simulink model "_LongLatDriveline"  (R2020b)
settings: Solver=FixedStepAuto  StartTime=0.0  StopTime=100  FixedStep=0.0005  RelTol=1e-3
InitFcn:
  | load('waypoints.mat');
  | VehicleObj = Simulink.data.dictionary.open('VehicleData.sldd');
  | %dDataSectObj = getSection(myDictionaryObj,'Design Data');
StopFcn:
  | Plot_LateralModelErrorControl;
values from neighbouring files (symbols this model uses):
  A_F = 2.341157    [VehicleData.sldd]
  C_af = 80000.0    [VehicleData.sldd]
  C_ar = 80000.0    [VehicleData.sldd]
  C_d = 0.24    [VehicleData.sldd]
  f = 0.01    [VehicleData.sldd]
  g = 9.81    [VehicleData.sldd]
  h_aero = 0.65    [VehicleData.sldd]
  h_gc = 0.65    [VehicleData.sldd]
  Iz = 2873.0    [VehicleData.sldd]
  lf = 1.1    [VehicleData.sldd]
  lr = 1.58    [VehicleData.sldd]
  m = 2238.932    [VehicleData.sldd]
  Nf = 2.0    [VehicleData.sldd]
  Nr = 2.0    [VehicleData.sldd]
  r_stat = 0.342    [VehicleData.sldd]
  r_w = 0.352    [VehicleData.sldd]
  rho = 1.225    [VehicleData.sldd]
  theta = 0.0    [VehicleData.sldd]
  transGear = 0.1027    [VehicleData.sldd]
  V_wind = 0.0    [VehicleData.sldd]
undefined symbols (not defined in the file or in its folder): sigbuilder_block
settings Model: DataDictionary=VehicleData.sldd  Creator=headl  LastModifiedBy=headl
settings DataIOCC: ReturnWorkspaceOutputs=off  DSMLoggingName=datalog
settings DebuggingCC: SignalRangeChecking=warning
settings SFSimCC: CustomCodeUndefinedFunction=UseInterfaceOnly

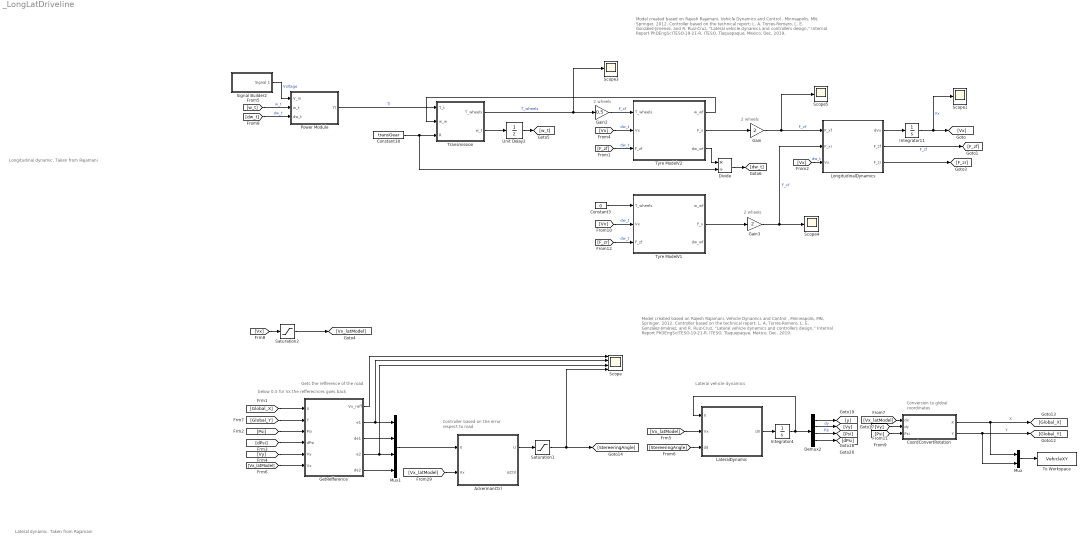
== system _LongLatDriveline ==
  note: below 0.5 for Vx the refferecnces goes back
  note: 2 wheels
  note: Model created based on
      | Rajesh Rajamani, Vehicle Dynamics and Control , Minneapolis, MN, Springer, 2012.
      |
      | Controller based on the technical report:
      | L. A. Torres-Romero, L. E. González-Jiménez, and R. Ruiz-Cruz, “Lateral vehicle dynamics and controllers design,” Internal Report PhDEngScITESO-19-21-R, ITESO, Tlaquepaque, Mexico, Dec. 2019.
  note: Lateral dynamic. Taken from Rajamani
  note: Conversion to global
      | coordinates
  note: Gets the refference of the road
  note: Controller based on the error
      | respect to road
  note: Lateral vehicle dynamics
  note: Longitudinal dynamic. Taken from Rajamani
  note: Model created based on
      | Rajesh Rajamani, Vehicle Dynamics and Control , Minneapolis, MN, Springer, 2012.
      |
      | Controller based on the technical report:
      | L. A. Torres-Romero, L. E. González-Jiménez, and R. Ruiz-Cruz, “Lateral vehicle dynamics and controllers design,” Internal Report PhDEngScITESO-19-21-R, ITESO, Tlaquepaque, Mexico, Dec. 2019.
  note: 2 wheels
  note: 2 wheels
  AckermanCtrl : MATLAB Function  TreatAsAtomicUnit=on
  Constant3 : Constant  Value=0
  Constant30 : Constant  Value=transGear
  CoordConvertRotation : Subsystem
  Demux2 : Demux
  Divide : Product  Inputs=*/
  Gain : Gain  Gain=2
  Gain2 : Gain  Gain=0.5
  Gain3 : Gain  Gain=2
  GetRefference : MATLAB Function  TreatAsAtomicUnit=on
  Integrator11 : Integrator
  Integrator4 : Integrator  InitialCondition=[0;0;-1.574;0.0423]
  LateralDynamic : MATLAB Function  TreatAsAtomicUnit=on
  LongitudinalDynamics : MATLAB Function  TreatAsAtomicUnit=on
  Mux : Mux  Inputs=2
  Mux1 : Mux
  Power Module : Subsystem  Variant=on  VariantControlMode=label  LabelModeActiveChoice=BLDC_Motor
  Saturation1 : Saturate  UpperLimit=pi/4  LowerLimit=-pi/4
  Saturation2 : Saturate  UpperLimit=1000000000  LowerLimit=0.5
  Scope : Scope  NumInputPorts=4
  Scope{1,3..5} (4 alike) : Scope
  Signal Builder2 : Subsystem  Tag=STV Subsys  LoadFcn=sigbuilder_block('load');  StartFcn=sigbuilder_block('start');  StopFcn=sigbuilder_block('stop');  ClipboardFcn=sigbuilder_block('clipboard');  mask(Sigbuilder block){tuvar=[0:10]}
      mask help: Simulink:masks:SigbuilderBlock_MD
      mask init:
      | if ~strcmp(get_param(bdroot(gcbh),'SimulationStatus'),'stopped') tuvar = sigbuilder_block('maskInit'); end
      settings: CopyFcn=sigbuilder_block('copy');  DeleteFcn=sigbuilder_block('delete');  ModelCloseFcn=sigbuilder_block('modelClose');  PreSaveFcn=sigbuilder_block('preSave');  PauseFcn=sigbuilder_block('pause');  ContinueFcn=sigbuilder_block('continue');  NameChangeFcn=sigbuilder_block('namechange');  OpenFcn=sigbuilder_block('open',[5.4 102.6 1141.2 483.6 ]);  CloseFcn=sigbuilder_block('close');
      mask Display: plot(0, 0, 100, 100,[2, 2, 32, 32, 2], [68, 8, 8, 68, 68],[32, 2], [38, 38], [32, 19, 2],[53, 60, 44], [32, 17, 17, 2],[16, 16, 31, 31]);txt = getActiveGroup(gcbh);text(2, 100, txt,'verticalAlignment', 'top');
  To Workspace : ToWorkspace  VariableName=VehicleXY  SampleTime=-1
  Transmission : MATLAB Function  TreatAsAtomicUnit=on
  Tyre ModelV1 : Subsystem
      mask Display: image('D:\Users\headl\MATLAB Drive\20_Control\SimulinkModels\VehicleModelV3\images\tire.png'); % Use "Edit Image" on toolstrip to change.
  Tyre ModelV2 : Subsystem
      mask Display: image('D:\Users\headl\MATLAB Drive\20_Control\SimulinkModels\VehicleModelV3\images\tire.png'); % Use "Edit Image" on toolstrip to change.
  Unit Delay2 : UnitDelay  SampleTime=-1  HasFrameUpgradeWarning=on
  wires:
  Demux2/1 -> [y]
  LateralDynamic/1(dX) -> Integrator4/1
  [Vx_latModel] -> CoordConvertRotation/1(dx)
  Integrator4/1 -> Demux2/1, LateralDynamic/1(X)
  [Vy] -> CoordConvertRotation/2(dy)
  Demux2/2 -> [Vy]  "dy"
  Demux2/4 -> [dPsi]
  Demux2/3 -> [Psi]  "Psi"
  [StereeringAngle] -> LateralDynamic/3(dd)
  [Psi] -> CoordConvertRotation/3(Psi)
  CoordConvertRotation/2(Y) -> Mux/2, [Global_Y]  "Y"
  CoordConvertRotation/1(X) -> Mux/1, [Global_X]  "X"
  [Vx_latModel] -> AckermanCtrl/2(Vx)
  Mux1/1 -> AckermanCtrl/1(X)
  Mux/1 -> To Workspace/1
  [Global_X] -> GetRefference/1(X)
  [Global_Y] -> GetRefference/2(Y)
  [Psi] -> GetRefference/3(Psi)
  [dPsi] -> GetRefference/4(dPsi)
  [Vy] -> GetRefference/5(Vy)
  [Vx_latModel] -> GetRefference/6(Vx)
  GetRefference/2(e1) -> Scope/2, Mux1/1
  GetRefference/3(de1) -> Mux1/2
  GetRefference/4(e2) -> Scope/3, Mux1/3
  GetRefference/5(de2) -> Mux1/4
  GetRefference/1(Vx_reff) -> Scope/1
  Divide/1 -> [dw_t]
  Transmission/2(w_t) -> Unit Delay2/1
  Constant30/1 -> Transmission/3(R), Divide/2
  Unit Delay2/1 -> [w_t]
  AckermanCtrl/1(U) -> Saturation1/1
  Saturation1/1 -> Scope/4, [StereeringAngle]
  Tyre ModelV2/3(dw_wf) -> Divide/1
  Tyre ModelV2/2(F_x) -> Gain/1
  Gain/1 -> Scope5/1, LongitudinalDynamics/1(F_xf)  "F_xf"
  [Vx] -> Tyre ModelV2/2(Vx)  "dw_t"
  [F_zf] -> Tyre ModelV2/3(F_zf)  "dw_t"
  Tyre ModelV2/1(w_wf) -> Transmission/2(w_w)
  [dw_t] -> Power Module/3(dw_t)  "dw_t"
  [w_t] -> Power Module/2(w_t)  "w_t"
  Signal Builder2/1(Signal 1) -> Power Module/1(V_in)  "Voltage"
  LongitudinalDynamics/1(dVx) -> Integrator11/1
  Transmission/1(T_wheels) -> Scope3/1, Gain2/1  "T_wheels"
  [Vx] -> LongitudinalDynamics/3(Vx)  "dw_t"
  Integrator11/1 -> Scope1/1, [Vx]  "Vx"
  [Vx_latModel] -> LateralDynamic/2(Vx)
  [Vx] -> Saturation2/1
  Saturation2/1 -> [Vx_latModel]
  Gain2/1 -> Tyre ModelV2/1(T_wheels)  "F_xf"
  Constant3/1 -> Tyre ModelV1/1(T_wheels)
  [Vx] -> Tyre ModelV1/2(Vx)  "dw_t"
  [F_zr] -> Tyre ModelV1/3(F_zf)  "dw_t"
  Tyre ModelV1/2(F_x) -> Gain3/1
  Gain3/1 -> Scope4/1, LongitudinalDynamics/2(F_xr)  "F_xf"
  LongitudinalDynamics/2(F_zf) -> [F_zf]  "F_zf"
  LongitudinalDynamics/3(F_zr) -> [F_zr]
  Power Module/1(Tl) -> Transmission/1(T_t)  "Tl"

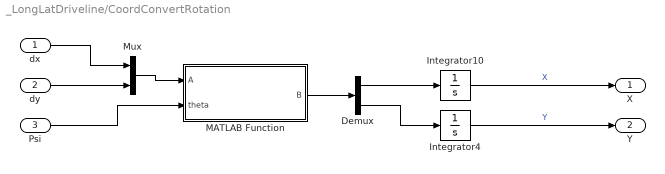
== system _LongLatDriveline/CoordConvertRotation ==
  dx : Inport
  dy : Inport  Port=2
  Psi : Inport  Port=3
  Demux : Demux  Outputs=2
  Integrator10 : Integrator  InitialCondition=-181.34188
  Integrator4 : Integrator  InitialCondition=78.53502
  MATLAB Function : MATLAB Function  TreatAsAtomicUnit=on
  Mux : Mux  Inputs=2
  X : Outport  VectorParamsAs1DForOutWhenUnconnected=off
  Y : Outport  Port=2  VectorParamsAs1DForOutWhenUnconnected=off
  wires:
  Integrator10/1 -> X/1  "X"
  Integrator4/1 -> Y/1  "Y"
  Psi/1 -> MATLAB Function/2(theta)
  dx/1 -> Mux/1
  dy/1 -> Mux/2
  Mux/1 -> MATLAB Function/1(A)
  MATLAB Function/1(B) -> Demux/1
  Demux/1 -> Integrator10/1
  Demux/2 -> Integrator4/1

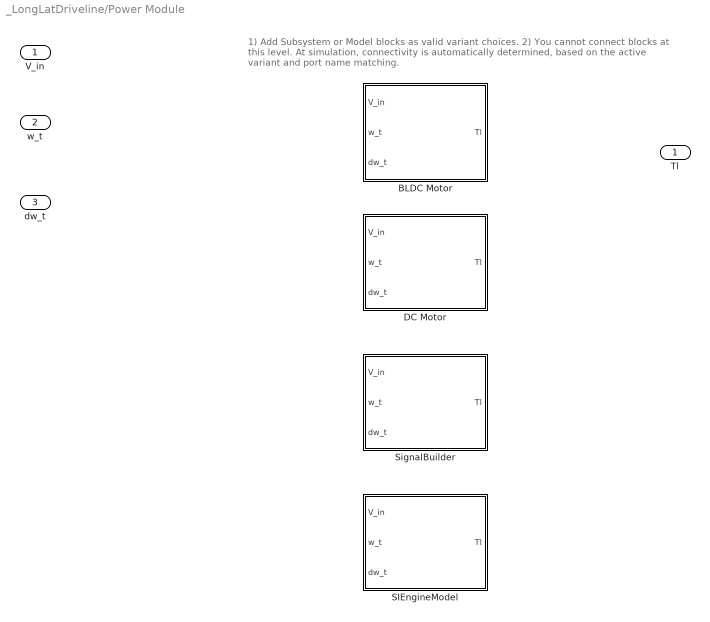
== system _LongLatDriveline/Power Module ==
  note: 1) Add Subsystem or Model blocks as valid variant choices.
      | 2) You cannot connect blocks at this level. At simulation, connectivity is automatically
      | determined, based on the active variant and port name matching.
  V_in : Inport
  w_t : Inport  Port=2
  dw_t : Inport  Port=3
  BLDC Motor : Subsystem  VariantControl=BLDC_Motor
      mask Display: image('D:\Users\headl\MATLAB Drive\20_Control\SimulinkModels\VehicleModelV4\images\BLDC.jpg'); % Use "Edit Image" on toolstrip to change.
  DC Motor : Subsystem  VariantControl=DC_Motor
  SIEngineModel : Subsystem  VariantControl=SI Engine
  SignalBuilder : Subsystem  VariantControl=Signal Bulder
  Tl : Outport

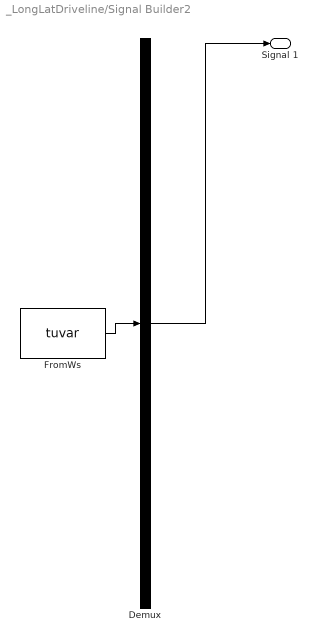
== system _LongLatDriveline/Signal Builder2 ==
  Demux : Demux  Tag=STV Demux  Outputs=1
      settings: DisplayOption=none
  FromWs : FromWorkspace  Tag=STV FromWs  VariableName=tuvar
      SigBuilderData=|
      | common.afterFinalStr = 'Extrapolate'
      | common.sampleTime = 0
      | dataSet.timeRange = [0 80]
      | dataSet.name = 'Group 1'
      | sbobj.Groups.Name = 'Group 1'
      | sbobj.Groups.Signals.Name = 'Signal 1'
      | sbobj.Groups.Signals.XData = [0 80]
      | sbobj.Groups.Signals.YData = [420 420]
      | sbobj.Groups.TimeRange = [0 80]
  Signal 1 : Outport  Tag=STV Outport  VectorParamsAs1DForOutWhenUnconnected=off
  wires:
  Demux/1 -> Signal 1/1
  FromWs/1 -> Demux/1

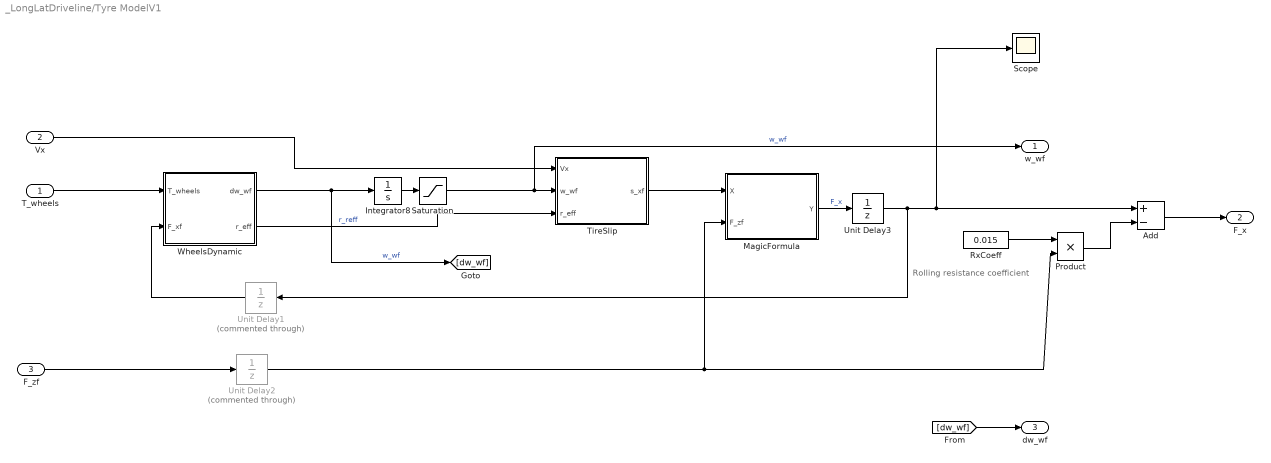
== system _LongLatDriveline/Tyre ModelV1 ==
  note: Rolling resistance coefficient
  T_wheels : Inport
  Vx : Inport  Port=2
  F_zf : Inport  Port=3
  Add : Sum  Inputs=+-
  Integrator8 : Integrator
  MagicFormula : MATLAB Function  TreatAsAtomicUnit=on
  Product : Product
  RxCoeff : Constant  Value=0.015
  Saturation : Saturate  UpperLimit=100000  LowerLimit=0
  Scope : Scope
  TireSlip : MATLAB Function  TreatAsAtomicUnit=on
  Unit Delay1 : UnitDelay  Commented=through  SampleTime=-1  HasFrameUpgradeWarning=on
  Unit Delay2 : UnitDelay  Commented=through  SampleTime=-1  HasFrameUpgradeWarning=on
  Unit Delay3 : UnitDelay  SampleTime=-1  HasFrameUpgradeWarning=on
  WheelsDynamic : MATLAB Function  TreatAsAtomicUnit=on
  w_wf : Outport
  F_x : Outport  Port=2
  dw_wf : Outport  Port=3
  wires:
  T_wheels/1 -> WheelsDynamic/1(T_wheels)
  Saturation/1 -> w_wf/1, TireSlip/2(w_wf)  "w_wf"
  WheelsDynamic/2(r_eff) -> TireSlip/3(r_eff)  "r_reff"
  MagicFormula/1(Y) -> Unit Delay3/1  "F_x"
  TireSlip/1(s_xf) -> MagicFormula/1(X)
  Integrator8/1 -> Saturation/1
  Vx/1 -> TireSlip/1(Vx)
  [dw_wf] -> dw_wf/1
  WheelsDynamic/1(dw_wf) -> [dw_wf], Integrator8/1  "w_wf"
  Add/1 -> F_x/1
  Product/1 -> Add/2
  RxCoeff/1 -> Product/1
  F_zf/1 -> Unit Delay2/1
  Unit Delay1/1 -> WheelsDynamic/2(F_xf)
  Unit Delay2/1 -> MagicFormula/2(F_zf), Product/2
  Unit Delay3/1 -> Unit Delay1/1, Add/1, Scope/1

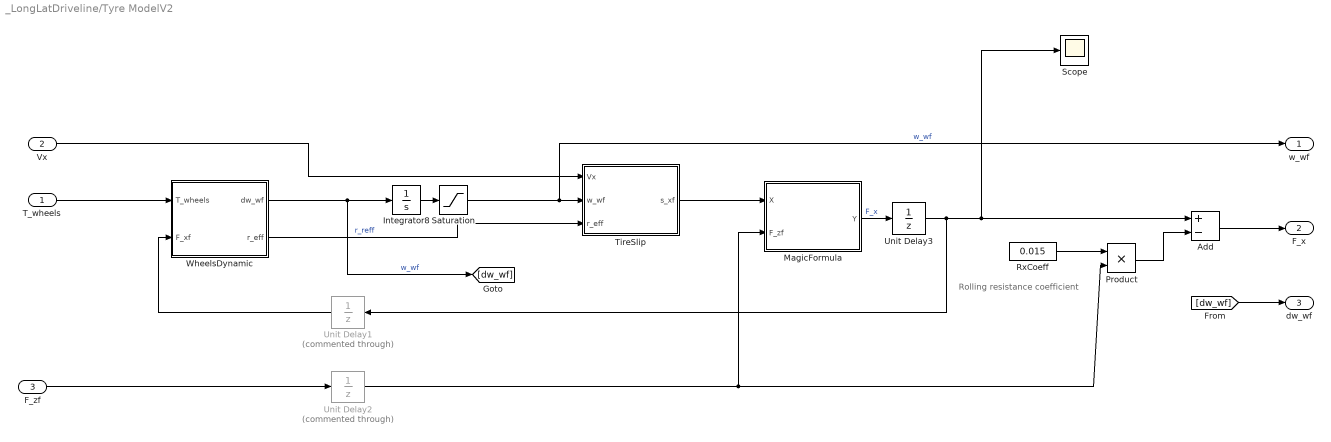
== system _LongLatDriveline/Tyre ModelV2 ==
  note: Rolling resistance coefficient
  T_wheels : Inport
  Vx : Inport  Port=2
  F_zf : Inport  Port=3
  Add : Sum  Inputs=+-
  Integrator8 : Integrator
  MagicFormula : MATLAB Function  TreatAsAtomicUnit=on
  Product : Product
  RxCoeff : Constant  Value=0.015
  Saturation : Saturate  UpperLimit=100000  LowerLimit=0
  Scope : Scope
  TireSlip : MATLAB Function  TreatAsAtomicUnit=on
  Unit Delay1 : UnitDelay  Commented=through  SampleTime=-1  HasFrameUpgradeWarning=on
  Unit Delay2 : UnitDelay  Commented=through  SampleTime=-1  HasFrameUpgradeWarning=on
  Unit Delay3 : UnitDelay  SampleTime=-1  HasFrameUpgradeWarning=on
  WheelsDynamic : MATLAB Function  TreatAsAtomicUnit=on
  w_wf : Outport
  F_x : Outport  Port=2
  dw_wf : Outport  Port=3
  wires:
  T_wheels/1 -> WheelsDynamic/1(T_wheels)
  Saturation/1 -> w_wf/1, TireSlip/2(w_wf)  "w_wf"
  WheelsDynamic/2(r_eff) -> TireSlip/3(r_eff)  "r_reff"
  MagicFormula/1(Y) -> Unit Delay3/1  "F_x"
  TireSlip/1(s_xf) -> MagicFormula/1(X)
  Integrator8/1 -> Saturation/1
  Vx/1 -> TireSlip/1(Vx)
  [dw_wf] -> dw_wf/1
  WheelsDynamic/1(dw_wf) -> [dw_wf], Integrator8/1  "w_wf"
  Add/1 -> F_x/1
  Product/1 -> Add/2
  RxCoeff/1 -> Product/1
  F_zf/1 -> Unit Delay2/1
  Unit Delay1/1 -> WheelsDynamic/2(F_xf)
  Unit Delay2/1 -> MagicFormula/2(F_zf), Product/2
  Unit Delay3/1 -> Unit Delay1/1, Add/1, Scope/1

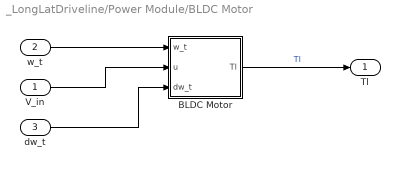
== system _LongLatDriveline/Power Module/BLDC Motor ==
  V_in : Inport
  w_t : Inport  Port=2
  dw_t : Inport  Port=3
  BLDC Motor : Subsystem
      mask Display: image('D:\Users\headl\MATLAB Drive\20_Control\SimulinkModels\VehicleModelV3\images\BLDC.jpg'); % Use "Edit Image" on toolstrip to change.
  Tl : Outport
  wires:
  w_t/1 -> BLDC Motor/1(w_t)
  V_in/1 -> BLDC Motor/2(u)
  dw_t/1 -> BLDC Motor/3(dw_t)
  BLDC Motor/1(Tl) -> Tl/1  "Tl"

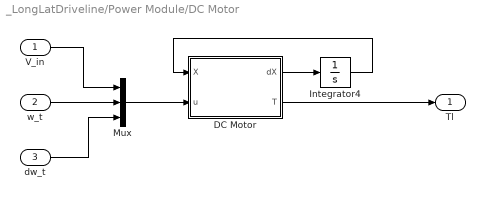
== system _LongLatDriveline/Power Module/DC Motor ==
  V_in : Inport
  w_t : Inport  Port=2
  dw_t : Inport  Port=3
  DC Motor : MATLAB Function  TreatAsAtomicUnit=on
  Integrator4 : Integrator
  Mux : Mux  Inputs=3
  Tl : Outport
  wires:
  dw_t/1 -> Mux/3
  DC Motor/1(dX) -> Integrator4/1
  Integrator4/1 -> DC Motor/1(X)
  Mux/1 -> DC Motor/2(u)
  w_t/1 -> Mux/2
  V_in/1 -> Mux/1
  DC Motor/2(T) -> Tl/1

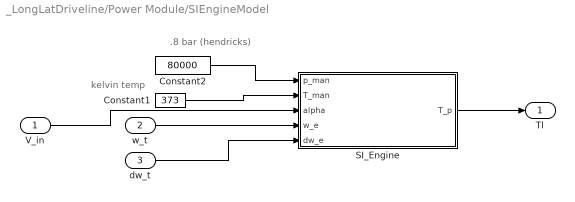
== system _LongLatDriveline/Power Module/SIEngineModel ==
  note: kelvin temp
  note: .8 bar (hendricks)
  V_in : Inport
  w_t : Inport  Port=2
  dw_t : Inport  Port=3
  Constant1 : Constant  Value=373
  Constant2 : Constant  Value=80000
  SI_Engine : Subsystem
  Tl : Outport
  wires:
  Constant2/1 -> SI_Engine/1(p_man)
  Constant1/1 -> SI_Engine/2(T_man)
  V_in/1 -> SI_Engine/3(alpha)
  w_t/1 -> SI_Engine/4(w_e)
  dw_t/1 -> SI_Engine/5(dw_e)
  SI_Engine/1(T_p) -> Tl/1

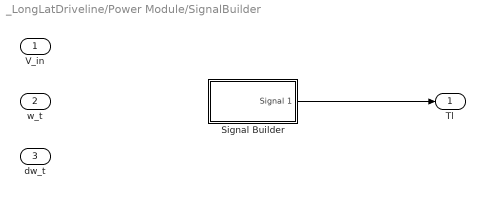
== system _LongLatDriveline/Power Module/SignalBuilder ==
  V_in : Inport
  w_t : Inport  Port=2
  dw_t : Inport  Port=3
  Signal Builder : Subsystem  Tag=STV Subsys  LoadFcn=sigbuilder_block('load');  StartFcn=sigbuilder_block('start');  StopFcn=sigbuilder_block('stop');  ClipboardFcn=sigbuilder_block('clipboard');  mask(Sigbuilder block){tuvar=[0:10]}
      mask help: Simulink:masks:SigbuilderBlock_MD
      mask init:
      | if ~strcmp(get_param(bdroot(gcbh),'SimulationStatus'),'stopped') tuvar = sigbuilder_block('maskInit'); end
      settings: CopyFcn=sigbuilder_block('copy');  DeleteFcn=sigbuilder_block('delete');  ModelCloseFcn=sigbuilder_block('modelClose');  PreSaveFcn=sigbuilder_block('preSave');  PauseFcn=sigbuilder_block('pause');  ContinueFcn=sigbuilder_block('continue');  NameChangeFcn=sigbuilder_block('namechange');  OpenFcn=sigbuilder_block('open',[437.6 199.2 550.4 400 ]);  CloseFcn=sigbuilder_block('close');
      mask Display: plot(0, 0, 100, 100,[2, 2, 32, 32, 2], [68, 8, 8, 68, 68],[32, 2], [38, 38], [32, 19, 2],[53, 60, 44], [32, 17, 17, 2],[16, 16, 31, 31]);txt = getActiveGroup(gcbh);text(2, 100, txt,'verticalAlignment', 'top');
  Tl : Outport
  wires:
  Signal Builder/1(Signal 1) -> Tl/1

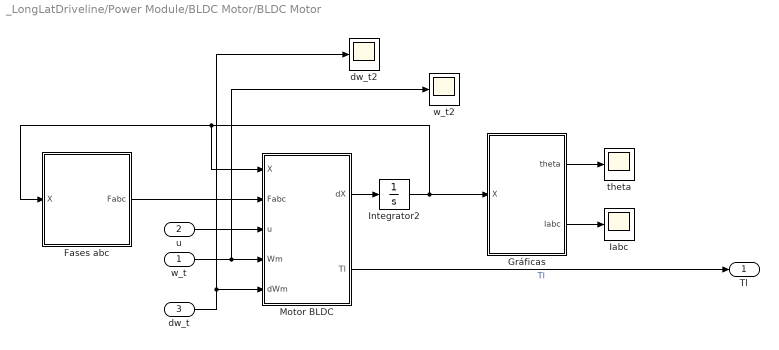
== system _LongLatDriveline/Power Module/BLDC Motor/BLDC Motor ==
  w_t : Inport
  u : Inport  Port=2
  dw_t : Inport  Port=3
  Fases abc : MATLAB Function  TreatAsAtomicUnit=on
  Gráficas : MATLAB Function  TreatAsAtomicUnit=on
  Iabc : Scope
  Integrator2 : Integrator  InitialCondition=[0 0 0 0]
  Motor BLDC : MATLAB Function  TreatAsAtomicUnit=on
  dw_t2 : Scope
  theta : Scope
  w_t2 : Scope
  Tl : Outport
  wires:
  dw_t/1 -> dw_t2/1, Motor BLDC/5(dWm)
  Integrator2/1 -> Gráficas/1(X), Motor BLDC/1(X), Fases abc/1(X)
  w_t/1 -> w_t2/1, Motor BLDC/4(Wm)
  Fases abc/1(Fabc) -> Motor BLDC/2(Fabc)
  Gráficas/2(Iabc) -> Iabc/1
  Motor BLDC/1(dX) -> Integrator2/1
  Gráficas/1(theta) -> theta/1
  Motor BLDC/2(Tl) -> Tl/1  "Tl"
  u/1 -> Motor BLDC/3(u)

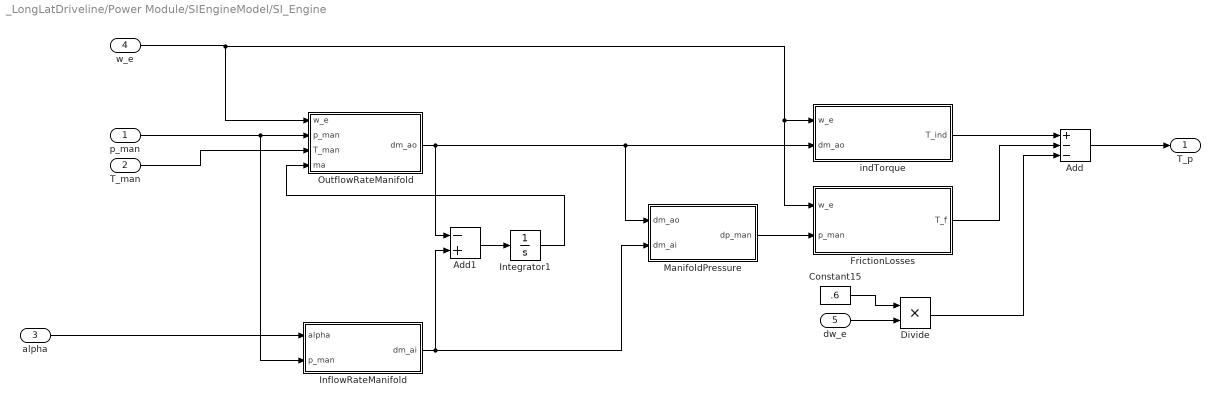
== system _LongLatDriveline/Power Module/SIEngineModel/SI_Engine ==
  p_man : Inport
  T_man : Inport  Port=2
  alpha : Inport  Port=3
  w_e : Inport  Port=4
  dw_e : Inport  Port=5
  Add : Sum  Inputs=+--
  Add1 : Sum  Inputs=-+
  Constant15 : Constant  Value=.6
  Divide : Product  Inputs=**
  FrictionLosses : MATLAB Function  TreatAsAtomicUnit=on
  InflowRateManifold : MATLAB Function  TreatAsAtomicUnit=on
  Integrator1 : Integrator
  ManifoldPressure : MATLAB Function  TreatAsAtomicUnit=on
  OutflowRateManifold : MATLAB Function  TreatAsAtomicUnit=on
  indTorque : MATLAB Function  TreatAsAtomicUnit=on
  T_p : Outport  VectorParamsAs1DForOutWhenUnconnected=off
  wires:
  ManifoldPressure/1(dp_man) -> FrictionLosses/2(p_man)
  InflowRateManifold/1(dm_ai) -> Add1/2, ManifoldPressure/2(dm_ai)
  OutflowRateManifold/1(dm_ao) -> Add1/1, ManifoldPressure/1(dm_ao), indTorque/2(dm_ao)
  indTorque/1(T_ind) -> Add/1
  p_man/1 -> InflowRateManifold/2(p_man), OutflowRateManifold/2(p_man)
  FrictionLosses/1(T_f) -> Add/2
  alpha/1 -> InflowRateManifold/1(alpha)
  Add1/1 -> Integrator1/1
  Integrator1/1 -> OutflowRateManifold/4(ma)
  T_man/1 -> OutflowRateManifold/3(T_man)
  w_e/1 -> FrictionLosses/1(w_e), indTorque/1(w_e), OutflowRateManifold/1(w_e)
  Constant15/1 -> Divide/1
  dw_e/1 -> Divide/2
  Divide/1 -> Add/3
  Add/1 -> T_p/1

== system _LongLatDriveline/Power Module/SignalBuilder/Signal Builder ==
  Demux : Demux  Tag=STV Demux  Outputs=1
      settings: DisplayOption=none
  FromWs : FromWorkspace  Tag=STV FromWs  VariableName=tuvar
      SigBuilderData=|
      | common.afterFinalStr = 'Extrapolate'
      | common.sampleTime = 0
      | dataSet.timeRange = [0 150]
      | dataSet.name = 'Group 1'
      | sbobj.Groups.Name = 'Group 1'
      | sbobj.Groups.Signals.Name = 'Signal 1'
      | sbobj.Groups.Signals.XData = [0 150]
      | sbobj.Groups.Signals.YData = [50 50]
      | sbobj.Groups.TimeRange = [0 150]
  Signal 1 : Outport  Tag=STV Outport
  wires:
  Demux/1 -> Signal 1/1
  FromWs/1 -> Demux/1

== matlab function _LongLatDriveline/AckermanCtrl ==
  data: U output size=1; X input; Vx input; isCtrl output size=1; C_af parameter; g parameter; C_ar parameter; lf parameter; lr parameter; Iz parameter; m parameter
% ******************* Lateral dynamic controller *********************
%*********************************************************************
% Author: L.Arturo Torres-Romero
% Date: 22-10-2020
% This controller controlls the direction of a car, based in the dynamics
% described  in the next link and using the Ackerman formulation: 
% https://www.researchgate.net/publication/340166902_LATERAL_VEHICLE_DYNAMICS_AND_CONTROLLERS_DESIGN
%******************* PARAMETERS DESCRIPTIONS **********************
%******************************************************************
% m: vehicle mass
% g: gravity
% C_af : Cornering  stiffness  of  front  wheels.
% C_ar : Cornering  stiffness  of  rear  wheels.
% lf : distance fron the center of gravity to the front wheel axis.
% lr : distance fron the center of gravity to the rear wheel axis.
% Iz : this is the momentum of inertia of the vehicle respect the z axis.
%******************************************************************
%******************* INPUTS DESCRIPTIONS **************************
%******************************************************************
% X:   (column vector)[e1;de1;e2;de2] states of the state space of 
%       the system that includes the errors as follows:
%      e1  : is the lateral position error respect the road.
%      de1 : derivative of e1.
%      e2  : is the yaw angle error with respect the road. 
%      de2 : derivarive of the e2.
% Vx: Logitudinal velocity.

%******************************************************************
% ******************* OUTPUTS DESCRIPTIONS ************************
%******************************************************************
% U: control coutput in radians. Angle of the frontal wheels respect to the
%    longitudinal axis
% isCtrl: when true means that the matrix Mc has full rank, and hence, the
%         system is controllable
%******************************************************************

function [U,isCtrl] = AckermanLateralCtrl(X, Vx, C_af, g, C_ar, lf, lr, Iz, m) % pd polos deseados

%**************************************************
%******* Matrix A formulation *********************
A22 = -(2*C_af + 2*C_ar)/(m*Vx);
A23 = (2*C_af + 2*C_ar)/m;
A24 = (-2*C_af*lf + 2*C_ar*lr)/(m*Vx);
A42 = -(2*C_af*lf - 2*C_ar*lr)/(Iz*Vx);
A43 = (2*C_af*lf - 2*C_ar*lr)/Iz;
A44 = -(2*C_af*lf^2 + 2*C_ar*lr^2)/(Iz*Vx);

A = [0 1 0 0;0 A22 A23 A24;0 0 0 1;0 A42 A43 A44];
%**************************************************

%**************************************************
%******* Matrix B1 formulation ********************
B1_2 = 2*C_af/m;
B1_4 = 2*C_af*lf/Iz;

B1 = [0;B1_2;0;B1_4];
%***************************************************

%***************************************************
%******* Matrix B2 formulation *********************
B2_2 = -(2*C_af*lf - 2*C_ar*lr)/(m*Vx) - Vx;
B2_4 = -(2*C_af*lf^2 + 2*C_ar*lr^2)/(Iz*Vx);

B2 = [0;B2_2;0;B2_4];
%***************************************************


%***************************************************
%******* Matrix B3 formulation *********************
B3 = [0;g;0;0];
%***************************************************


%***************************************************
%******* Verification of controllability and output 
% calculation of the controller
%**************************************************
ctrlVal = 0;
Mc = [B1 A*B1 A^2*B1 A^3*B1];
rankVal = rank(Mc);
    if rankVal < size(A,1)
        %disp('Not completely state controllable');
        isCtrl = 0;
        ctrlVal = 0;
    else
        %disp('Completely state controllable');
        isCtrl = 1;
        % Pole placement
        Pd =[-5-3i -5+3i -7 -10];
        %Pd =[-2 -2 -2 -2];

        H = (A- Pd(1)*eye(4)) * (A- Pd(2)*eye(4)) * (A- Pd(3)*eye(4)) * (A- Pd(4)*eye(4));

        %ackerman formula
        K = [0 0 0 1]*Mc^-1*H;
        ctrlVal = -K*X;  
    end


U = real(ctrlVal);

== matlab function _LongLatDriveline/Tyre ModelV1/WheelsDynamic ==
  data: T_wheels input; dw_wf output; r_eff output; F_xf input; r_w parameter; r_stat parameter
% ******************* Wheel inertia dynamics *********************
%****************************************************************
% BASED ON 
% Rajesh Rajamani, Vehicle Dynamics and Control, Minneapolis, MN, Springer, 2012.
%Chapter 4.2.4
% r_eff = effective radius of the wheel
% F_xf = longitudinal tire force from the front wheels



function [dw_wf, r_eff]= fcn(T_wheels,F_xf, r_w, r_stat)

%r_w = 0.352; % radius of the tire. Pirelli Sottozero 3 P245/45WR19
%r_stat = 0.342; % static vertical deflection of the tire
alpha = acos(r_stat/r_w);
r_eff = (alpha*r_w)/alpha;


I_w = .9; % TODO define this
dw_wf = (T_wheels -(r_eff*F_xf))/I_w;

== matlab function _LongLatDriveline/Tyre ModelV2/MagicFormula ==
  data: X input; Y output; F_zf input
%BASED ON
%Massimo Guiggiani, The Science of Vehicle Dynamics, Pisa, Italy, Springer Netherlands, 2014.
%Chapter 2.12
%The values of the MF were obtained from the graph in fig. 2.22

function Y = XTireForce(X, F_zf) 
% B stiffness factor
% C shape factor
% D peak value
% E curvature factor
% Sh horizontal shift
% Sv vertical shift

Sh = 0;% Sh horizontal shift
Sv = 0; %vertical shift

D = 3; % ym, maximum value Experimental from graph
C = 1.5;
B = 20;
E = 0;

x = X-Sh;
gamma = C*atan(B*x-E*(B*x-atan(B*x)));
y = F_zf*D*sin(gamma);
Y = (y - Sv);

== matlab function _LongLatDriveline/Tyre ModelV2/TireSlip ==
  data: Vx input; s_xf output; w_wf input; r_eff input
%BASED ON
%Rajesh Rajamani, Vehicle Dynamics and Control, Minneapolis, MN, Springer, 2012.
%Chapter 4.1.2

function s_xf = XTireSlip(Vx,w_wf,r_eff) 

if Vx == 0
   s_xf = 0.1 * sign(w_wf);   
else
   s_xf = (r_eff*w_wf -Vx)/abs(Vx); % acceleration
end

if s_xf > 1
   %s_xf = 1; 
end

== matlab function _LongLatDriveline/Power Module/SIEngineModel/SI_Engine/FrictionLosses ==
  data: w_e input; T_f output; p_man input
function T_f = fcn(w_e, p_man)
% According Heywood 98 friction loss = .97 +0.15*(N/1000)+  0.05(N/1000)^2
% Where N is RPM. here it is converted to rad/s



a0 = 4.559432e-6;
a1 = 0.009550;
a2 = .97;
b0 = 0;
b1 = 0;




T_f = abs(a0*w_e^2 + a1*w_e + a2 + b0*w_e*p_man + b1*p_man);a1*w_e + a2 + b0*w_e*p_man + b1*p_man;

== matlab function _LongLatDriveline/Power Module/BLDC Motor/BLDC Motor/Motor BLDC ==
  data: X input; dX output; Fabc input; u input; Wm input; dWm input; Tl output
function [dX,Tl] = fcn(X,Fabc,u,Wm,dWm)
Iabc = X(2:4);
R = 0.7;
L = 0.005;%0.00272-0.0015; %=L-Lm
J = 0.000284;
b = 0.02;
P = 4;
maxTl = 400; % max torque of the motor
Lambda = 0.105;

Vabc = u*Fabc;

Eabc = Lambda*Wm*Fabc;
dTheta = P*Wm/2;

if Wm > 0.01
Te = (Iabc'*Eabc)/Wm;
Tl = Te-b*Wm-J*dWm;
else
Tl  = maxTl;
end

if Tl > maxTl
Tl = maxTl;   
end

dIabc = (-R*Iabc - Eabc + Vabc)/L;

dX = [dTheta;dIabc];
end

== matlab function _LongLatDriveline/Power Module/DC Motor/DC Motor ==
  data: X input; dX output; u input size=3; T output
function [dX, T]= fcn(X,u)
ia = X(1);
Va = u(1); wm =u(2); dwm =u(3);

MaxT = 800;

Ra = 0.193;
La = 0.00383;
Jm = 0.6;
Bm = 2.632177;
Kb = 2.332232;
KT = 2.1717;

A1 = -Ra/La;
B1 = [1/La -Kb/La 0];
C1 = KT;
D1 = [0 -Bm -Jm];

dX = A1*X + B1*u;
T = C1*X + D1*u;

if T > MaxT
    T = MaxT;
end
if T < 0
    T = 0;
end

end

== matlab function _LongLatDriveline/Power Module/SIEngineModel/SI_Engine/InflowRateManifold ==
  data: alpha input; dm_ai output; p_man input
function dm_ai = fcn(alpha,p_man)

% Max  Automotive Powertrain Modeling for Control (D.Cho and J. K. Hedrick)
MAX = 0.1843; % Kg/s constant dependent on the size of the throttle body and is equalto the maximum possible intake airflow rate.
alpha_p = 0.05; %the minimum throttle angle seen by the engine.
pc = 0.5283; % critical pressure ratio
p_amb =101325; % pressure of 1 atm in Pa
p_r = p_man/p_amb;

if p_r <= pc
PRI = 1; % p_r <= pc Sonic
else
PRI = sqrt(1-((p_r-pc)/(1-pc))^2); % P_r > pc   chocked
end

TC = 1-cos(alpha-alpha_p);
dm_ai = MAX * TC * PRI;

== matlab function _LongLatDriveline/Power Module/SIEngineModel/SI_Engine/ManifoldPressure ==
  data: dm_ao input; dm_ai input; dp_man output
function dp_man = fcn(dm_ao,dm_ai)
R = 8.314472; % (J/(K*mol)) ideal gas constant.
T_man = 60; % intake manifold temperature.
V_man = 1; % intake manifold volume

dp_man = (R*T_man*(dm_ai-dm_ao))/V_man;

== matlab function _LongLatDriveline/LongitudinalDynamics ==
  data: F_xf input; dVx output; F_xr input; Vx input; rho parameter; g parameter; A_F parameter; C_d parameter; f parameter; m parameter; V_wind parameter; theta parameter; F_zf output; F_zr output; h_aero parameter; h_gc parameter; lf parameter; lr parameter; Nf parameter; Nr parameter
% BASED ON
% Rajesh Rajamani, Vehicle Dynamics and Control, Minneapolis, MN, Springer, 2012.
%Chapter 4.1

function [dVx,F_zf, F_zr] = LongitudinalDynamics(F_xf,F_xr,Vx, rho, g, A_F, C_d, f, m, V_wind, theta, h_aero, h_gc, lf, lr, Nf, Nr)
% m = 2238.932; % TESLA model S P85D
% g = 9.81;
% theta = 0;
% A_F = 2.341157; % Fontal area of the vehicle. TESLA model S P85D
% C_d  =0.24; %Ford Focus Aerodynamic drag coeficient. TESLA model S P85D
% rho = 1.225;  %(kg/m^3) Air density
% f = 0.01; % varies from 0.01 to 0.04
% V_wind = 0;
% Nf, Nr Number of wheels in front and rear axles

F_aero = (1/2)*rho*C_d*A_F*(Vx+V_wind)^2;

dVx = (F_xf + F_xr - F_aero - m*g*sin(theta))/m;

F_zf = (-F_aero*h_aero -m*dVx*h_gc -m*g*h_gc*sin(theta) +m*g*lr*cos(theta))/(Nf*(lr+lf));
F_zr = ( F_aero*h_aero +m*dVx*h_gc +m*g*h_gc*sin(theta) +m*g*lf*cos(theta))/(Nr*(lr+lf));

== matlab function _LongLatDriveline/Power Module/SIEngineModel/SI_Engine/OutflowRateManifold ==
  data: w_e input; dm_ao output; p_man input; T_man input; ma input
function dm_ao = fcn(w_e, p_man, T_man,ma)
Vd = 0.0038; %displacement volume of the engine cylinders
R = 8.31446261815324; %constant used in ideal gas law for intake manifold

%volumetric efficiency

% Automotive Powertrain Modeling for Control (D.Cho and J. K. Hedrick)
eta_vol = (24.5*w_e -3.1e4)*ma^2 + (-1.167*w_e+222)*ma +(8.1e-4*w_e+0.352);
%eta_vol = 0.9;

dm_ao = ((eta_vol*w_e*Vd)/(4*pi))*(p_man/(R*T_man));

== matlab function _LongLatDriveline/Power Module/SIEngineModel/SI_Engine/indTorque ==
  data: w_e input; T_ind output; dm_ao input
function T_ind = fcn(w_e, dm_ao)
% dm_ao: air mass flow rate out of the intake manifold and into the cylinder
% dm_f:  is the mass fuel rate into the cylinders 
H_u = 46000000; % fuel energy constant. look in other sources 44-46 MJ/kg found as (Gasoline heating value)
h_i = 0.45; % Thermal efficiency multiplier. Otto engine value.   from (Hendricks and Sorenson, 1990)
lambda = 1; % air/fuel equivalence ratio
L_th = 14.67; % stoichiometric air/fuel mass ratio for gasoline.


dm_f = dm_ao/(L_th*lambda);

if w_e ~= 0
T_ind = (H_u*h_i*dm_f)/w_e;   
else
T_ind = (H_u*h_i*dm_f)/0.01;    
end

== matlab function _LongLatDriveline/Tyre ModelV2/WheelsDynamic ==
  data: T_wheels input; dw_wf output; r_eff output; F_xf input; r_w parameter; r_stat parameter
% ******************* Wheel inertia dynamics *********************
%****************************************************************
% BASED ON 
% Rajesh Rajamani, Vehicle Dynamics and Control, Minneapolis, MN, Springer, 2012.
%Chapter 4.2.4
% r_eff = effective radius of the wheel
% F_xf = longitudinal tire force from the front wheels



function [dw_wf, r_eff]= fcn(T_wheels,F_xf, r_w, r_stat)

%r_w = 0.352; % radius of the tire. Pirelli Sottozero 3 P245/45WR19
%r_stat = 0.342; % static vertical deflection of the tire
alpha = acos(r_stat/r_w);
r_eff = (alpha*r_w)/alpha;


I_w = .9; % TODO define this
dw_wf = (T_wheels -(r_eff*F_xf))/I_w;

== matlab function _LongLatDriveline/Transmission ==
  data: T_wheels output; T_t input; w_t output; w_w input; R input
% ***************** Transmission ******************
% *************************************************
% BASED ON
% Rajesh Rajamani, Vehicle Dynamics and Control, Minneapolis, MN, Springer, 2012.
% Chapter 4.2.2
% T_wheels = wheels torque
% w_w = wheels angular speed
% R = gear ratio of transmission
%**************************************************

function [T_wheels, w_t]= fcn(T_t,w_w,R)

T_wheels = T_t/R;
w_t = w_w/R;
% itneed to be implemented "during change"

== matlab function _LongLatDriveline/CoordConvertRotation/MATLAB Function ==
  data: A input; B output; theta input
function B = RotateVector(A, theta)
B = [0;0];
R = [cos(theta) -sin(theta); sin(theta) cos(theta)];

B = R*A;

== matlab function _LongLatDriveline/Tyre ModelV1/MagicFormula ==
  data: X input; Y output; F_zf input
%BASED ON
%Massimo Guiggiani, The Science of Vehicle Dynamics, Pisa, Italy, Springer Netherlands, 2014.
%Chapter 2.12
%The values of the MF were obtained from the graph in fig. 2.22

function Y = XTireForce(X, F_zf) 
% B stiffness factor
% C shape factor
% D peak value
% E curvature factor
% Sh horizontal shift
% Sv vertical shift

Sh = 0;% Sh horizontal shift
Sv = 0; %vertical shift

D = 3; % ym, maximum value Experimental from graph
C = 1.5;
B = 20;
E = 0;

x = X-Sh;
gamma = C*atan(B*x-E*(B*x-atan(B*x)));
y = F_zf*D*sin(gamma);
Y = (y - Sv);

== matlab function _LongLatDriveline/Power Module/BLDC Motor/BLDC Motor/Fases abc ==
  data: X input; Fabc output
function Fabc = fcn(X)
    theta = mod(X(1),2*pi);
    
    if (0<=theta)&&(theta<(pi/6))
        Fa = (6/pi)*theta;
    elseif ((pi/6)<=theta)&&(theta<(5*pi/6))
        Fa = 1;
    elseif ((5*pi/6<=theta))&&(theta<(7*pi/6))
        Fa = (6/pi)*(pi-theta);
    elseif ((7*pi/6)<=theta)&&(theta<(11*pi/6))
        Fa = -1;
    elseif ((11*pi/6)<=theta)&&(theta<(2*pi))
        Fa = (6/pi)*(theta-2*pi);
    else
        Fa = NaN;
    end
    
    if (0<=theta)&&(theta<(3*pi/6))
        Fb = -1;
    elseif ((3*pi/6)<=theta)&&(theta<(5*pi/6))
        Fb = (6/pi)*(theta-(2*pi)/3);
    elseif ((5*pi/6)<=theta)&&(theta<(9*pi/6))
        Fb = 1;
    elseif ((9*pi/6)<=theta)&&(theta<(11*pi/6))
        Fb = (6/pi)*(-theta+(5*pi)/3);
    elseif ((11*pi/6)<=theta)&&(theta<(2*pi))
        Fb = -1;
    else
        Fb = NaN;
    end
    
    if (0<=theta)&&(theta<(pi/6))
        Fc = 1;
    elseif ((pi/6)<=theta)&&(theta<(3*pi/6))
        Fc = (6/pi)*(pi/3-theta);
    elseif ((3*pi/6)<=theta)&&(theta<(7*pi/6))
        Fc = -1;
    elseif ((7*pi/6)<=theta)&&(theta<(9*pi/6))
        Fc = (6/pi)*(theta-(4*pi)/3);
    elseif ((9*pi/6)<=theta)&&(theta<(2*pi))
        Fc = 1;
    else
        Fc = NaN; 
    end
    
    Fabc = [Fa;Fb;Fc];
end

== matlab function _LongLatDriveline/Power Module/BLDC Motor/BLDC Motor/Gráficas ==
  data: X input; theta output; Iabc output
function [theta,Iabc] = DEMUX(X)
theta = X(1);Iabc = X(2:4);

== matlab function _LongLatDriveline/GetRefference ==
  data: Vx_reff output; e1 output size=1; X input size=1; Y input double size=1; racetrackwaypoints parameter; de1 output; e2 output; de2 output; Psi input; dPsi input; Vy input; Vx input
% ******************* GetRefference *********************
%*********************************************************************
% Author: L.Arturo Torres-Romero
% Date: 22-10-2020
% BICYCLE MODEL OF LATERAL VEHICLE DYNAMICS
% Based on Rajamani chapter 2.3 page 30 and  in the next publication with
% the controller
% https://www.researchgate.net/publication/340166902_LATERAL_VEHICLE_DYNAMICS_AND_CONTROLLERS_DESIGN
% This block gets the errors required for the controller of the steering wheel that is based in the error respect the road.
% In this case the road is specified as a list of points (waypoints) in the array racetrackwaypoints
%******************************************************************
%******************* INPUTS DESCRIPTIONS **************************
%******************************************************************
% X:   Global coordinate X of the C.G. of the vehicle 
% Y:   Global coordinate X of the C.G. of the vehicle
% racetrackwaypoints: array with a list of waypoints of the road [X Y]
% Psi: Is the yaw angle respect to the inertial global system
% dPsi: Angular velocity of the yaw angle.
% Vy: Lateral velocity
% Vx: Longitudinal velocity
%******************************************************************
% ******************* OUTPUTS DESCRIPTIONS ************************
%******************************************************************
% e1  : is the lateral position error respect the road.
% de1 : derivative of e1.
% e2  : is the yaw angle error with respect the road. 
% de2 : derivarive of the e2.

function [Vx_reff,e1,de1,e2,de2] = GetReff(X,Y,racetrackwaypoints, Psi,dPsi, Vy, Vx) 

PQ = [X,Y]; % current Intertial position of vehicle
P = racetrackwaypoints(:,1:2); % List of waypoints column1 = X coord.  column2 = Y coord. Column 3 = Vx for reference
[k,D] = knnsearch(P,PQ); % locate the closest waypoint to the vehicle. k = index, D = distance
k = k(1);


% here I take 3 points: the closest, one behind, one in front.
P_road1 = P(k-1,:);
P_road2 = P(k,:);
P_road3 = P(k+1,:);
Vx_reff = racetrackwaypoints(k,3);
Vx_reff = Vx_reff(1);

F = atan2( (P(k+5,2)-P(k,2)),(P(k+5,1)-P(k,1))); % Obtaining the road orientation
psi_des = F(1);

P_veh = PQ - P_road2;

%B = [P(k,1);P(k,2)];
% Convert from intertial coordinates system to body fixed system. C.G. as
% center and rotated Psi degrees.
M_Rot = [cos(psi_des) -sin(psi_des); sin(psi_des) cos(psi_des)];
P_veh = P_veh*M_Rot;

e1 = P_veh(2); % error e1

e2 = Psi - psi_des; % error e2

de1 = Vy + Vx*(e2); % derivative of e1


% Obtainig the radius of imaginary circle of the curve
Xc = [P_road1(1);P_road2(1);P_road3(1)];
Yc = [P_road1(2);P_road2(2);P_road3(2)];
[xc,yc,R,a] = circfit(Xc,Yc);
C = [xc yc];
C = (C-P_road2)*M_Rot;
xc = C(1);
yc = C(2);
R = R*sign(yc);


%in streight line, the radius falls into singularity. here is detected
%and solved with a minimum
eval = ~isfinite(R);
if eval
 R = 100000; % in case of NaN define a straight line as an arc of circle of R very big.
end

dPsi_des = Vx/R; % derivative of orientation refference
de2 = dPsi - dPsi_des; % derivative of e2

end

== matlab function _LongLatDriveline/LateralDynamic ==
  data: dX output; X input; Vx input; dd input; C_af parameter; C_ar parameter; lf parameter; lr parameter; Iz parameter; m parameter
% ******************* Lateral dynamic controller *********************
%*********************************************************************
% Author: L.Arturo Torres-Romero
% Date: 22-10-2020
% BICYCLE MODEL OF LATERAL VEHICLE DYNAMICS
% Based on Rajamani chapter 2.3 page 30 and  in the next publication with
% the controller
% https://www.researchgate.net/publication/340166902_LATERAL_VEHICLE_DYNAMICS_AND_CONTROLLERS_DESIGN
%******************* PARAMETERS DESCRIPTIONS **********************
%******************************************************************
% m: vehicle mass
% g: gravity
% C_af : Cornering  stiffness  of  front  wheels.
% C_ar : Cornering  stiffness  of  rear  wheels.
% lf : distance fron the center of gravity to the front wheel axis.
% lr : distance fron the center of gravity to the rear wheel axis.
% Iz : this is the momentum of inertia of the vehicle respect the z axis.
%******************************************************************
%******************* INPUTS DESCRIPTIONS **************************
%******************************************************************
% X:   (column vector)[y;dy;Psi;dPsi] states of the state space of 
%       the system that includes:
%      y  : Radius of the curve that the car is performing.
%      dy : Lateral velocity.
%      Psi  : Is the yaw angle respect to the inertial global system
%      dPsi : Angular velocity of the yaw angle.
% Vx: Logitudinal velocity.

function dX = DynamicBicycleModel(X,Vx,dd, C_af, C_ar, lf, lr, Iz, m) % pd polos deseados
dX = [0;0;0;0];
y = X(1);
dy = X(2);
Psi = X(3);
dPsi = X(4);


A22 = -(2*C_af+2*C_ar)/(m*Vx);
A24 = -Vx- (2*C_af*lf-2*C_ar*lr)/(m*Vx);
A42 = -(2*lf*C_af-2*lr*C_ar)/(Iz*Vx);
A44 = -(2*lf^2*C_af + 2*lr^2*C_ar)/(Iz*Vx);

B21 = 2*C_af/m;
B41 = 2*lf*C_af/Iz;

A = [0 1 0 0;0 A22 0 A24;0 0 0 1;0 A42 0 A44];
B = [0;B21;0;B41];

dX= A*X(1:4) + B*dd; 

end

== matlab function _LongLatDriveline/Tyre ModelV1/TireSlip ==
  data: Vx input; s_xf output; w_wf input; r_eff input
%BASED ON
%Rajesh Rajamani, Vehicle Dynamics and Control, Minneapolis, MN, Springer, 2012.
%Chapter 4.1.2

function s_xf = XTireSlip(Vx,w_wf,r_eff) 

if Vx == 0
   s_xf = 0.1 * sign(w_wf);   
else
   s_xf = (r_eff*w_wf -Vx)/abs(Vx); % acceleration
end

if s_xf > 1
   %s_xf = 1; 
end
